simulink model "ProcessFlowRateModel_IMHRC2014v3"  (Simulink 7.9)
settings: Solver=VariableStepDiscrete  StartTime=0.0  StopTime=100.0  RelTol=1e-3
libraries: simeventslib x14
(part 2 of 2)

== system ProcessFlowRateModel_IMHRC2014v3/Pallet_STORE/Calculate_OUTFlow ==
  Calculate_OUTFlow : MATLAB Function  TreatAsAtomicUnit=on
  Entity Combiner : EntityCombiner  NumberInputPorts=2
  Entity Sink : EntitySink
  Entity Splitter : EntitySplitter  NumberOutputPorts=2
  FIFO Queue : FIFOQueue  Capacity=inf
  Get Attribute : GetAttribute  AttributeName=UoH|Quantity|OUTFlow  AttributeMissing=Error|Error|Error  AttributeDefaultValue=1|1|1  AttributeTreatAsVector=1|1|1  AttributeSendTiming=After entity departure|After entity departure|After entity departure  EvaluatedDefaultAttributeValue={[];[];[]}
      settings: OutputPortMap=o1,o2,o3
  Set Attribute : SetAttribute  AttributeName=OUTFlow  AttributeFrom=Signal port  EvaluatedAttributeValue={[]}
  Single Server : SingleServer  ServiceTime=0
  FlowRecord_IN : PMIOPort  Port=1  Side=Left
  FlowRecord_OUT : PMIOPort  Port=2  Side=Left
  OUTFlow_Signal : PMIOPort  Port=3  Side=Right
  wires:
  Get Attribute/1 -> Calculate_OUTFlow/1(UoH)
  Calculate_OUTFlow/1(OUTFlow_return) -> Set Attribute/1
  Get Attribute/2 -> Calculate_OUTFlow/2(Quantity)
  Get Attribute/3 -> Calculate_OUTFlow/3(OUTFlow)
  connections:
  Entity Combiner/RConn1 -- Get Attribute/LConn1
  Set Attribute/RConn1 -- Entity Splitter/LConn1
  Get Attribute/RConn1 -- Single Server/LConn1
  Single Server/RConn1 -- Set Attribute/LConn1
  FlowRecord_OUT/RConn1 -- Entity Splitter/RConn1
  FlowRecord_IN/RConn1 -- Entity Combiner/LConn1
  OUTFlow_Signal/RConn1 -- FIFO Queue/LConn1
  FIFO Queue/RConn1 -- Entity Combiner/LConn2
  Entity Splitter/RConn2 -- Entity Sink/LConn1

== system ProcessFlowRateModel_IMHRC2014v3/Pallet_STORE/FlowRecord ==
  Discrete Event Signal to Workspace : simeventslib/SimEvents Sinks/Discrete Event Signal to Workspace  VariableName=INFlow_Metric_PalletStore  SaveFormat=Structure With Time  isMonitorOnly=off  isRecordIC=off
  Discrete Event Signal to Workspace1 : simeventslib/SimEvents Sinks/Discrete Event Signal to Workspace  VariableName=OUTFlow_Metric_PalletStore  SaveFormat=Structure With Time  isMonitorOnly=off  isRecordIC=off
  FIFO Queue : FIFOQueue
  FlowRecord : TimeBasedFunctionCallGenerator  EventGenerationMode=Only at simulation start
  Get Attribute : GetAttribute  AttributeName=OUTFlow|INFlow  AttributeMissing=Error|Error  AttributeDefaultValue=1|1  AttributeTreatAsVector=1|1  AttributeSendTiming=After entity departure|After entity departure  EvaluatedDefaultAttributeValue={[];[]}
      settings: OutputPortMap=o1,o2
  Initialize_FlowRecord : SetAttribute  AttributeName=INFlow|OUTFlow  AttributeFrom=Dialog|Dialog  AttributeValue=[0 0 0 0 0]|[0 0 0 0 0]  AttributeTreatAsVector=1|1  EvaluatedAttributeValue={[0 0 0 0 0];[0 0 0 0 0]}
  New_FlowRecord : EventBasedEntityGenerator  GenerateEntitiesUpon=Function call from port fcn
  Output Switch : OutputSwitch  NumberOutputPorts=2
  Path Combiner1 : PathCombiner
  TO_INFlow : PMIOPort  Port=1  Side=Right
  TO_OUTFlow : PMIOPort  Port=2  Side=Left
  FROM_INFlow : PMIOPort  Port=3  Side=Right
  FROM_OUTFlow : PMIOPort  Port=4  Side=Left
  wires:
  FlowRecord/1 -> New_FlowRecord/1
  Get Attribute/2 -> Discrete Event Signal to Workspace/1
  Get Attribute/1 -> Discrete Event Signal to Workspace1/1
  connections:
  Output Switch/LConn1 -- FIFO Queue/RConn1
  New_FlowRecord/RConn1 -- Initialize_FlowRecord/LConn1
  Initialize_FlowRecord/RConn1 -- Path Combiner1/LConn1
  TO_INFlow/RConn1 -- Output Switch/RConn1
  TO_OUTFlow/RConn1 -- Output Switch/RConn2
  FROM_INFlow/RConn1 -- Path Combiner1/LConn2
  FROM_OUTFlow/RConn1 -- Path Combiner1/LConn3
  Path Combiner1/RConn1 -- Get Attribute/LConn1
  Get Attribute/RConn1 -- FIFO Queue/LConn1

== system ProcessFlowRateModel_IMHRC2014v3/Pallet_STORE/STORE ==
  Entity Sink : EntitySink
  FROM_STORE : Replicate  NumberOutputPorts=2
  InventoryRecord : Subsystem
  Message2Flow : Subsystem
  Message_Queue : FIFOQueue
  TO_STORE : Replicate  NumberOutputPorts=2
  Update_InventoryRecord_INFlow : Subsystem
  Update_InventoryRecord_OUTFlow : Subsystem
  Flow_IN : PMIOPort  Port=1  Side=Left
  Message_IN : PMIOPort  Port=2  Side=Left
  Flow_OUT : PMIOPort  Port=3  Side=Right
  Message_OUT : PMIOPort  Port=4  Side=Right
  connections:
  InventoryRecord/RConn1 -- Update_InventoryRecord_INFlow/RConn1
  Update_InventoryRecord_INFlow/RConn2 -- InventoryRecord/RConn2
  Flow_IN/RConn1 -- TO_STORE/LConn1
  TO_STORE/RConn1 -- Update_InventoryRecord_INFlow/LConn1
  TO_STORE/RConn2 -- Entity Sink/LConn1
  Message2Flow/RConn1 -- FROM_STORE/LConn1
  FROM_STORE/RConn2 -- Flow_OUT/RConn1
  Update_InventoryRecord_OUTFlow/LConn1 -- FROM_STORE/RConn1
  InventoryRecord/LConn1 -- Update_InventoryRecord_OUTFlow/RConn1
  InventoryRecord/LConn2 -- Update_InventoryRecord_OUTFlow/RConn2
  Message_IN/RConn1 -- Message_Queue/LConn1
  Message_Queue/RConn1 -- Message2Flow/LConn1

== system ProcessFlowRateModel_IMHRC2014v3/Parcel_OA/Calculate_INFlow ==
  Calculate_INFlow : MATLAB Function  TreatAsAtomicUnit=on
  Entity Combiner : EntityCombiner  NumberInputPorts=2
  Entity Sink : EntitySink
  Entity Splitter : EntitySplitter  NumberOutputPorts=2
  FIFO Queue : FIFOQueue  Capacity=inf
  Get Attribute : GetAttribute  AttributeName=UoH|Quantity|INFlow  AttributeMissing=Error|Error|Error  AttributeDefaultValue=1|1|1  AttributeTreatAsVector=1|1|1  AttributeSendTiming=After entity departure|After entity departure|After entity departure  EvaluatedDefaultAttributeValue={[];[];[]}
      settings: OutputPortMap=o1,o2,o3
  Set Attribute : SetAttribute  AttributeName=INFlow  AttributeFrom=Signal port  EvaluatedAttributeValue={[]}
  Single Server : SingleServer  ServiceTime=0
  FlowRecord_IN : PMIOPort  Port=1  Side=Right
  FlowRecord_OUT : PMIOPort  Port=2  Side=Right
  INFlow_Signal : PMIOPort  Port=3  Side=Left
  wires:
  Get Attribute/1 -> Calculate_INFlow/1(UoH)
  Calculate_INFlow/1(INFlow_return) -> Set Attribute/1
  Get Attribute/2 -> Calculate_INFlow/2(Quantity)
  Get Attribute/3 -> Calculate_INFlow/3(INFlow)
  connections:
  Entity Combiner/RConn1 -- Get Attribute/LConn1
  Set Attribute/RConn1 -- Entity Splitter/LConn1
  Get Attribute/RConn1 -- Single Server/LConn1
  Single Server/RConn1 -- Set Attribute/LConn1
  FlowRecord_OUT/RConn1 -- Entity Splitter/RConn1
  FlowRecord_IN/RConn1 -- Entity Combiner/LConn1
  Entity Splitter/RConn2 -- Entity Sink/LConn1
  INFlow_Signal/RConn1 -- FIFO Queue/LConn1
  FIFO Queue/RConn1 -- Entity Combiner/LConn2

== system ProcessFlowRateModel_IMHRC2014v3/Parcel_OA/Calculate_OUTFlow ==
  Calculate_OUTFlow : MATLAB Function  TreatAsAtomicUnit=on
  Entity Combiner : EntityCombiner  NumberInputPorts=2
  Entity Sink : EntitySink
  Entity Splitter : EntitySplitter  NumberOutputPorts=2
  FIFO Queue : FIFOQueue  Capacity=inf
  Get Attribute : GetAttribute  AttributeName=UoH|Quantity|OUTFlow  AttributeMissing=Error|Error|Error  AttributeDefaultValue=1|1|1  AttributeTreatAsVector=1|1|1  AttributeSendTiming=After entity departure|After entity departure|After entity departure  EvaluatedDefaultAttributeValue={[];[];[]}
      settings: OutputPortMap=o1,o2,o3
  Set Attribute : SetAttribute  AttributeName=OUTFlow  AttributeFrom=Signal port  EvaluatedAttributeValue={[]}
  Single Server : SingleServer  ServiceTime=0
  FlowRecord_IN : PMIOPort  Port=1  Side=Left
  FlowRecord_OUT : PMIOPort  Port=2  Side=Left
  OUTFlow_Signal : PMIOPort  Port=3  Side=Right
  wires:
  Get Attribute/1 -> Calculate_OUTFlow/1(UoH)
  Calculate_OUTFlow/1(OUTFlow_return) -> Set Attribute/1
  Get Attribute/2 -> Calculate_OUTFlow/2(Quantity)
  Get Attribute/3 -> Calculate_OUTFlow/3(OUTFlow)
  connections:
  Entity Combiner/RConn1 -- Get Attribute/LConn1
  Set Attribute/RConn1 -- Entity Splitter/LConn1
  Get Attribute/RConn1 -- Single Server/LConn1
  Single Server/RConn1 -- Set Attribute/LConn1
  FlowRecord_OUT/RConn1 -- Entity Splitter/RConn1
  FlowRecord_IN/RConn1 -- Entity Combiner/LConn1
  OUTFlow_Signal/RConn1 -- FIFO Queue/LConn1
  FIFO Queue/RConn1 -- Entity Combiner/LConn2
  Entity Splitter/RConn2 -- Entity Sink/LConn1

== system ProcessFlowRateModel_IMHRC2014v3/Parcel_OA/FRN_Process ==
  FIFO Queue1 : FIFOQueue
  N-Server : NServer  NumberOfServers=inf  ServiceTime=0
  Flow_IN : PMIOPort  Port=1  Side=Left
  Message_IN : PMIOPort  Port=2  Side=Left
  Flow_OUT : PMIOPort  Port=3  Side=Right
  Message_OUT : PMIOPort  Port=4  Side=Right
  connections:
  FIFO Queue1/RConn1 -- N-Server/LConn1
  Flow_IN/RConn1 -- FIFO Queue1/LConn1
  Flow_OUT/RConn1 -- N-Server/RConn1
  Message_OUT/RConn1 -- Message_IN/RConn1

== system ProcessFlowRateModel_IMHRC2014v3/Parcel_OA/FlowRecord ==
  Discrete Event Signal to Workspace : simeventslib/SimEvents Sinks/Discrete Event Signal to Workspace  VariableName=INFlow_Metric  SaveFormat=Structure With Time  isMonitorOnly=off  isRecordIC=off
  Discrete Event Signal to Workspace1 : simeventslib/SimEvents Sinks/Discrete Event Signal to Workspace  VariableName=OUTFlow_Metric  SaveFormat=Structure With Time  isMonitorOnly=off  isRecordIC=off
  FIFO Queue : FIFOQueue
  FlowRecord : TimeBasedFunctionCallGenerator  EventGenerationMode=Only at simulation start
  Get Attribute : GetAttribute  AttributeName=OUTFlow|INFlow  AttributeMissing=Error|Error  AttributeDefaultValue=1|1  AttributeTreatAsVector=1|1  AttributeSendTiming=After entity departure|After entity departure  EvaluatedDefaultAttributeValue={[];[]}
      settings: OutputPortMap=o1,o2
  Initialize_FlowRecord : SetAttribute  AttributeName=INFlow|OUTFlow  AttributeFrom=Dialog|Dialog  AttributeValue=[0 0 0 0 0]|[0 0 0 0 0]  AttributeTreatAsVector=1|1  EvaluatedAttributeValue={[0 0 0 0 0];[0 0 0 0 0]}
  New_FlowRecord : EventBasedEntityGenerator  GenerateEntitiesUpon=Function call from port fcn
  Output Switch : OutputSwitch  NumberOutputPorts=2
  Path Combiner1 : PathCombiner
  TO_INFlow : PMIOPort  Port=1  Side=Right
  TO_OUTFlow : PMIOPort  Port=2  Side=Left
  FROM_INFlow : PMIOPort  Port=3  Side=Right
  FROM_OUTFlow : PMIOPort  Port=4  Side=Left
  wires:
  FlowRecord/1 -> New_FlowRecord/1
  Get Attribute/2 -> Discrete Event Signal to Workspace/1
  Get Attribute/1 -> Discrete Event Signal to Workspace1/1
  connections:
  Output Switch/LConn1 -- FIFO Queue/RConn1
  New_FlowRecord/RConn1 -- Initialize_FlowRecord/LConn1
  Initialize_FlowRecord/RConn1 -- Path Combiner1/LConn1
  TO_INFlow/RConn1 -- Output Switch/RConn1
  TO_OUTFlow/RConn1 -- Output Switch/RConn2
  FROM_INFlow/RConn1 -- Path Combiner1/LConn2
  FROM_OUTFlow/RConn1 -- Path Combiner1/LConn3
  Path Combiner1/RConn1 -- Get Attribute/LConn1
  Get Attribute/RConn1 -- FIFO Queue/LConn1

== system ProcessFlowRateModel_IMHRC2014v3/Parcel_SHIP/OrderFamily_Parcel_SOURCE ==
  Carton_Quantity1 : EventBasedRandomNumber  Distribution=Discrete uniform  minUnid=1  maxUnid=15  numValueUnid=15  valueVecDisc=[1 2 3]  probVecDisc=[0.5 0.35 0.15]  Seed=38014
  Pallet_Source1 : TimeBasedEntityGenerator
  Set_Pallet1 : SetAttribute  AttributeName=UoH|CartonQuantity|Quantity  AttributeFrom=Dialog|Signal port|Dialog  AttributeValue=1|1|1  AttributeTreatAsVector=1|1|1  EvaluatedAttributeValue={1;[];1}
      settings: InputPortMap=u1
  Conn1 : PMIOPort  Port=1  Side=Right
  wires:
  Carton_Quantity1/1 -> Set_Pallet1/1
  connections:
  Pallet_Source1/RConn1 -- Set_Pallet1/LConn1
  Conn1/RConn1 -- Set_Pallet1/RConn1

== system ProcessFlowRateModel_IMHRC2014v3/Each_STORE/STORE/InventoryRecord ==
  Discrete Event Signal to Workspace : simeventslib/SimEvents Sinks/Discrete Event Signal to Workspace  VariableName=Net_Inventory_PalletStore  SaveFormat=Structure With Time  isMonitorOnly=off  isRecordIC=off
  FIFO Queue : FIFOQueue
  Get Attribute : GetAttribute  AttributeName=Net_Inventory  EvaluatedDefaultAttributeValue={[]}
      settings: OutputPortMap=o1
  Initialize_FlowRecord : SetAttribute  AttributeName=Net_Inventory  AttributeValue=[0 0 0 0 0]  EvaluatedAttributeValue={[0 0 0 0 0]}
  InventoryRecord : TimeBasedFunctionCallGenerator  EventGenerationMode=Only at simulation start
  New_InventoryRecord : EventBasedEntityGenerator  GenerateEntitiesUpon=Function call from port fcn
  Output Switch : OutputSwitch  NumberOutputPorts=2
  Path Combiner : PathCombiner
  TO_INFlow : PMIOPort  Port=1  Side=Right
  TO_OUTFlow : PMIOPort  Port=2  Side=Left
  FROM_INFlow : PMIOPort  Port=3  Side=Right
  FROM_OUTFlow : PMIOPort  Port=4  Side=Left
  wires:
  InventoryRecord/1 -> New_InventoryRecord/1
  Get Attribute/1 -> Discrete Event Signal to Workspace/1
  connections:
  Output Switch/LConn1 -- FIFO Queue/RConn1
  New_InventoryRecord/RConn1 -- Initialize_FlowRecord/LConn1
  Initialize_FlowRecord/RConn1 -- Path Combiner/LConn1
  TO_INFlow/RConn1 -- Output Switch/RConn1
  TO_OUTFlow/RConn1 -- Output Switch/RConn2
  FROM_INFlow/RConn1 -- Path Combiner/LConn2
  FROM_OUTFlow/RConn1 -- Path Combiner/LConn3
  Path Combiner/RConn1 -- Get Attribute/LConn1
  Get Attribute/RConn1 -- FIFO Queue/LConn1

== system ProcessFlowRateModel_IMHRC2014v3/Each_STORE/STORE/Message2Flow ==
  Entity Departure Function-Call Generator : EntityDepartureFunctionCallGenerator
  Generate_Flow_Entity : EventBasedEntityGenerator  GenerateEntitiesUpon=Function call from port fcn
  Get_Order_Attribute : GetAttribute  AttributeName=UoH|Quantity  AttributeMissing=Error|Error  AttributeDefaultValue=1|1  AttributeTreatAsVector=1|1  AttributeSendTiming=After entity departure|After entity departure  EvaluatedDefaultAttributeValue={[];[]}
      settings: OutputPortMap=o1,o2
  Message_Sink : EntitySink
  Set_Flow_Attribute : SetAttribute  AttributeName=UoH|Quantity  AttributeFrom=Signal port|Signal port  AttributeValue=1|1  AttributeTreatAsVector=1|1  EvaluatedAttributeValue={[];[]}
      settings: InputPortMap=u0,u1
  Single Server : SingleServer  ServiceTime=0
  Message_IN : PMIOPort  Port=1  Side=Left
  Flow_OUT : PMIOPort  Port=2  Side=Right
  wires:
  Entity Departure Function-Call Generator/1 -> Generate_Flow_Entity/1
  Get_Order_Attribute/1 -> Set_Flow_Attribute/1
  Get_Order_Attribute/2 -> Set_Flow_Attribute/2
  connections:
  Get_Order_Attribute/RConn1 -- Entity Departure Function-Call Generator/LConn1
  Entity Departure Function-Call Generator/RConn1 -- Message_Sink/LConn1
  Generate_Flow_Entity/RConn1 -- Single Server/LConn1
  Single Server/RConn1 -- Set_Flow_Attribute/LConn1
  Message_IN/RConn1 -- Get_Order_Attribute/LConn1
  Flow_OUT/RConn1 -- Set_Flow_Attribute/RConn1

== system ProcessFlowRateModel_IMHRC2014v3/Each_STORE/STORE/Update_InventoryRecord_INFlow ==
  Calculate_Inventory : MATLAB Function  TreatAsAtomicUnit=on
  Entity Combiner : EntityCombiner  NumberInputPorts=2
  Entity Sink : EntitySink
  Entity Splitter : EntitySplitter  NumberOutputPorts=2
  FIFO Queue : FIFOQueue  Capacity=inf
  Get Attribute : GetAttribute  AttributeName=UoH|Quantity|Net_Inventory  AttributeMissing=Error|Error|Error  AttributeDefaultValue=1|1|1  AttributeTreatAsVector=1|1|1  AttributeSendTiming=After entity departure|After entity departure|After entity departure  EvaluatedDefaultAttributeValue={[];[];[]}
      settings: OutputPortMap=o1,o2,o3
  Set Attribute : SetAttribute  AttributeName=Net_Inventory  AttributeFrom=Signal port  EvaluatedAttributeValue={[]}
  Single Server : SingleServer  ServiceTime=0
  InventoryRecord_IN : PMIOPort  Port=1  Side=Right
  InventoryRecord_OUT : PMIOPort  Port=2  Side=Right
  Signal_IN : PMIOPort  Port=3  Side=Left
  wires:
  Get Attribute/1 -> Calculate_Inventory/1(UoH)
  Calculate_Inventory/1(Net_Inventory1) -> Set Attribute/1
  Get Attribute/2 -> Calculate_Inventory/2(Quantity)
  Get Attribute/3 -> Calculate_Inventory/3(Net_Inventory)
  connections:
  Entity Combiner/RConn1 -- Get Attribute/LConn1
  Set Attribute/RConn1 -- Entity Splitter/LConn1
  Get Attribute/RConn1 -- Single Server/LConn1
  Single Server/RConn1 -- Set Attribute/LConn1
  InventoryRecord_OUT/RConn1 -- Entity Splitter/RConn1
  InventoryRecord_IN/RConn1 -- Entity Combiner/LConn1
  Entity Splitter/RConn2 -- Entity Sink/LConn1
  Signal_IN/RConn1 -- FIFO Queue/LConn1
  FIFO Queue/RConn1 -- Entity Combiner/LConn2

== system ProcessFlowRateModel_IMHRC2014v3/Each_STORE/STORE/Update_InventoryRecord_OUTFlow ==
  Calculate_Inventory : MATLAB Function  TreatAsAtomicUnit=on
  Entity Combiner : EntityCombiner  NumberInputPorts=2
  Entity Sink : EntitySink
  Entity Splitter : EntitySplitter  NumberOutputPorts=2
  FIFO Queue : FIFOQueue  Capacity=inf
  Get Attribute : GetAttribute  AttributeName=UoH|Quantity|Net_Inventory  AttributeMissing=Error|Error|Error  AttributeDefaultValue=1|1|1  AttributeTreatAsVector=1|1|1  AttributeSendTiming=After entity departure|After entity departure|After entity departure  EvaluatedDefaultAttributeValue={[];[];[]}
      settings: OutputPortMap=o1,o2,o3
  Set Attribute : SetAttribute  AttributeName=Net_Inventory  AttributeFrom=Signal port  EvaluatedAttributeValue={[]}
  Single Server : SingleServer  ServiceTime=0
  InventoryRecord_IN : PMIOPort  Port=1  Side=Right
  InventoryRecord_OUT : PMIOPort  Port=2  Side=Right
  Signal_IN : PMIOPort  Port=3  Side=Left
  wires:
  Get Attribute/1 -> Calculate_Inventory/1(UoH)
  Calculate_Inventory/1(Net_Inventory1) -> Set Attribute/1
  Get Attribute/2 -> Calculate_Inventory/2(Quantity)
  Get Attribute/3 -> Calculate_Inventory/3(Net_Inventory)
  connections:
  Entity Combiner/RConn1 -- Get Attribute/LConn1
  Set Attribute/RConn1 -- Entity Splitter/LConn1
  Get Attribute/RConn1 -- Single Server/LConn1
  Single Server/RConn1 -- Set Attribute/LConn1
  InventoryRecord_OUT/RConn1 -- Entity Splitter/RConn1
  InventoryRecord_IN/RConn1 -- Entity Combiner/LConn1
  Entity Splitter/RConn2 -- Entity Sink/LConn1
  Signal_IN/RConn1 -- FIFO Queue/LConn1
  FIFO Queue/RConn1 -- Entity Combiner/LConn2

== system ProcessFlowRateModel_IMHRC2014v3/Pallet_STORE/STORE/InventoryRecord ==
  Discrete Event Signal to Workspace : simeventslib/SimEvents Sinks/Discrete Event Signal to Workspace  VariableName=Net_Inventory_PalletStore  SaveFormat=Structure With Time  isMonitorOnly=off  isRecordIC=off
  FIFO Queue : FIFOQueue
  Get Attribute : GetAttribute  AttributeName=Net_Inventory  EvaluatedDefaultAttributeValue={[]}
      settings: OutputPortMap=o1
  Initialize_FlowRecord : SetAttribute  AttributeName=Net_Inventory  AttributeValue=[0 0 0 0 0]  EvaluatedAttributeValue={[0 0 0 0 0]}
  InventoryRecord : TimeBasedFunctionCallGenerator  EventGenerationMode=Only at simulation start
  New_InventoryRecord : EventBasedEntityGenerator  GenerateEntitiesUpon=Function call from port fcn
  Output Switch : OutputSwitch  NumberOutputPorts=2
  Path Combiner : PathCombiner
  TO_INFlow : PMIOPort  Port=1  Side=Right
  TO_OUTFlow : PMIOPort  Port=2  Side=Left
  FROM_INFlow : PMIOPort  Port=3  Side=Right
  FROM_OUTFlow : PMIOPort  Port=4  Side=Left
  wires:
  InventoryRecord/1 -> New_InventoryRecord/1
  Get Attribute/1 -> Discrete Event Signal to Workspace/1
  connections:
  Output Switch/LConn1 -- FIFO Queue/RConn1
  New_InventoryRecord/RConn1 -- Initialize_FlowRecord/LConn1
  Initialize_FlowRecord/RConn1 -- Path Combiner/LConn1
  TO_INFlow/RConn1 -- Output Switch/RConn1
  TO_OUTFlow/RConn1 -- Output Switch/RConn2
  FROM_INFlow/RConn1 -- Path Combiner/LConn2
  FROM_OUTFlow/RConn1 -- Path Combiner/LConn3
  Path Combiner/RConn1 -- Get Attribute/LConn1
  Get Attribute/RConn1 -- FIFO Queue/LConn1

== system ProcessFlowRateModel_IMHRC2014v3/Pallet_STORE/STORE/Message2Flow ==
  Entity Departure Function-Call Generator : EntityDepartureFunctionCallGenerator
  Generate_Flow_Entity : EventBasedEntityGenerator  GenerateEntitiesUpon=Function call from port fcn
  Get_Order_Attribute : GetAttribute  AttributeName=UoH|Quantity  AttributeMissing=Error|Error  AttributeDefaultValue=1|1  AttributeTreatAsVector=1|1  AttributeSendTiming=After entity departure|After entity departure  EvaluatedDefaultAttributeValue={[];[]}
      settings: OutputPortMap=o1,o2
  Message_Sink : EntitySink
  Set_Flow_Attribute : SetAttribute  AttributeName=UoH|Quantity  AttributeFrom=Signal port|Signal port  AttributeValue=1|1  AttributeTreatAsVector=1|1  EvaluatedAttributeValue={[];[]}
      settings: InputPortMap=u0,u1
  Single Server : SingleServer  ServiceTime=0
  Message_IN : PMIOPort  Port=1  Side=Left
  Flow_OUT : PMIOPort  Port=2  Side=Right
  wires:
  Entity Departure Function-Call Generator/1 -> Generate_Flow_Entity/1
  Get_Order_Attribute/1 -> Set_Flow_Attribute/1
  Get_Order_Attribute/2 -> Set_Flow_Attribute/2
  connections:
  Get_Order_Attribute/RConn1 -- Entity Departure Function-Call Generator/LConn1
  Entity Departure Function-Call Generator/RConn1 -- Message_Sink/LConn1
  Generate_Flow_Entity/RConn1 -- Single Server/LConn1
  Single Server/RConn1 -- Set_Flow_Attribute/LConn1
  Message_IN/RConn1 -- Get_Order_Attribute/LConn1
  Flow_OUT/RConn1 -- Set_Flow_Attribute/RConn1

== system ProcessFlowRateModel_IMHRC2014v3/Pallet_STORE/STORE/Update_InventoryRecord_INFlow ==
  Calculate_Inventory : MATLAB Function  TreatAsAtomicUnit=on
  Entity Combiner : EntityCombiner  NumberInputPorts=2
  Entity Sink : EntitySink
  Entity Splitter : EntitySplitter  NumberOutputPorts=2
  FIFO Queue : FIFOQueue  Capacity=inf
  Get Attribute : GetAttribute  AttributeName=UoH|Quantity|Net_Inventory  AttributeMissing=Error|Error|Error  AttributeDefaultValue=1|1|1  AttributeTreatAsVector=1|1|1  AttributeSendTiming=After entity departure|After entity departure|After entity departure  EvaluatedDefaultAttributeValue={[];[];[]}
      settings: OutputPortMap=o1,o2,o3
  Set Attribute : SetAttribute  AttributeName=Net_Inventory  AttributeFrom=Signal port  EvaluatedAttributeValue={[]}
  Single Server : SingleServer  ServiceTime=0
  InventoryRecord_IN : PMIOPort  Port=1  Side=Right
  InventoryRecord_OUT : PMIOPort  Port=2  Side=Right
  Signal_IN : PMIOPort  Port=3  Side=Left
  wires:
  Get Attribute/1 -> Calculate_Inventory/1(UoH)
  Calculate_Inventory/1(Net_Inventory1) -> Set Attribute/1
  Get Attribute/2 -> Calculate_Inventory/2(Quantity)
  Get Attribute/3 -> Calculate_Inventory/3(Net_Inventory)
  connections:
  Entity Combiner/RConn1 -- Get Attribute/LConn1
  Set Attribute/RConn1 -- Entity Splitter/LConn1
  Get Attribute/RConn1 -- Single Server/LConn1
  Single Server/RConn1 -- Set Attribute/LConn1
  InventoryRecord_OUT/RConn1 -- Entity Splitter/RConn1
  InventoryRecord_IN/RConn1 -- Entity Combiner/LConn1
  Entity Splitter/RConn2 -- Entity Sink/LConn1
  Signal_IN/RConn1 -- FIFO Queue/LConn1
  FIFO Queue/RConn1 -- Entity Combiner/LConn2

== system ProcessFlowRateModel_IMHRC2014v3/Pallet_STORE/STORE/Update_InventoryRecord_OUTFlow ==
  Calculate_Inventory : MATLAB Function  TreatAsAtomicUnit=on
  Entity Combiner : EntityCombiner  NumberInputPorts=2
  Entity Sink : EntitySink
  Entity Splitter : EntitySplitter  NumberOutputPorts=2
  FIFO Queue : FIFOQueue  Capacity=inf
  Get Attribute : GetAttribute  AttributeName=UoH|Quantity|Net_Inventory  AttributeMissing=Error|Error|Error  AttributeDefaultValue=1|1|1  AttributeTreatAsVector=1|1|1  AttributeSendTiming=After entity departure|After entity departure|After entity departure  EvaluatedDefaultAttributeValue={[];[];[]}
      settings: OutputPortMap=o1,o2,o3
  Set Attribute : SetAttribute  AttributeName=Net_Inventory  AttributeFrom=Signal port  EvaluatedAttributeValue={[]}
  Single Server : SingleServer  ServiceTime=0
  InventoryRecord_IN : PMIOPort  Port=1  Side=Right
  InventoryRecord_OUT : PMIOPort  Port=2  Side=Right
  Signal_IN : PMIOPort  Port=3  Side=Left
  wires:
  Get Attribute/1 -> Calculate_Inventory/1(UoH)
  Calculate_Inventory/1(Net_Inventory1) -> Set Attribute/1
  Get Attribute/2 -> Calculate_Inventory/2(Quantity)
  Get Attribute/3 -> Calculate_Inventory/3(Net_Inventory)
  connections:
  Entity Combiner/RConn1 -- Get Attribute/LConn1
  Set Attribute/RConn1 -- Entity Splitter/LConn1
  Get Attribute/RConn1 -- Single Server/LConn1
  Single Server/RConn1 -- Set Attribute/LConn1
  InventoryRecord_OUT/RConn1 -- Entity Splitter/RConn1
  InventoryRecord_IN/RConn1 -- Entity Combiner/LConn1
  Entity Splitter/RConn2 -- Entity Sink/LConn1
  Signal_IN/RConn1 -- FIFO Queue/LConn1
  FIFO Queue/RConn1 -- Entity Combiner/LConn2

== matlab function LTL_OA/Calculate_INFlow/Calculate_INFlow ==
  data: UoH input double; INFlow_return output double; Quantity input double; INFlow input double
function INFlow_return  = Calculate_INFlow(UoH, Quantity, INFlow)
%#codegen

INFlow_return = INFlow;


if eq(UoH, 0) == 0
%test if parameters are initialized

    INFlow_return(UoH) = INFlow(UoH) + Quantity;
end

== matlab function LTL_OA/Calculate_OUTFlow/Calculate_OUTFlow ==
  data: UoH input double; OUTFlow_return output double; Quantity input double; OUTFlow input double
function OUTFlow_return  = Calculate_OUTFlow(UoH, Quantity, OUTFlow)
%#codegen

OUTFlow_return = OUTFlow;


if eq(UoH, 0) == 0
%test if parameters are initialized

    OUTFlow_return(UoH) = OUTFlow(UoH) + Quantity;
end

== matlab function Pallet_STORE/Calculate_INFlow/Calculate_INFlow ==
  data: UoH input double; INFlow_return output double; Quantity input double; INFlow input double
function INFlow_return  = Calculate_INFlow(UoH, Quantity, INFlow)
%#codegen

INFlow_return = INFlow;


if eq(UoH, 0) == 0
%test if parameters are initialized

    INFlow_return(UoH) = INFlow(UoH) + Quantity;
end

== matlab function Pallet_STORE/Calculate_OUTFlow/Calculate_OUTFlow ==
  data: UoH input double; OUTFlow_return output double; Quantity input double; OUTFlow input double
function OUTFlow_return  = Calculate_OUTFlow(UoH, Quantity, OUTFlow)
%#codegen

OUTFlow_return = OUTFlow;


if eq(UoH, 0) == 0
%test if parameters are initialized

    OUTFlow_return(UoH) = OUTFlow(UoH) + Quantity;
end

== matlab function Pallet_STORE/STORE/Update_InventoryRecord_INFlow/Calculate_Inventory ==
  data: UoH input double; Quantity input double; Net_Inventory input double; Net_Inventory1 output double
function Net_Inventory1  = Calculate_INFlow(UoH, Quantity, Net_Inventory)
%#codegen

Net_Inventory1 = Net_Inventory;


if eq(UoH, 0) == 0
%test if parameters are initialized

    Net_Inventory1(UoH) = Net_Inventory(UoH) + Quantity;
end

== matlab function Pallet_STORE/STORE/Update_InventoryRecord_OUTFlow/Calculate_Inventory ==
  data: UoH input double; Quantity input double; Net_Inventory input double; Net_Inventory1 output double
function Net_Inventory1  = Calculate_INFlow(UoH, Quantity, Net_Inventory)
%#codegen

Net_Inventory1 = Net_Inventory;


if eq(UoH, 0) == 0
%test if parameters are initialized

    Net_Inventory1(UoH) = Net_Inventory(UoH) - Quantity;
end

== matlab function MixedPallet_Assy/Calculate_INFlow/Calculate_INFlow ==
  data: UoH input double; INFlow_return output double; Quantity input double; INFlow input double
function INFlow_return  = Calculate_INFlow(UoH, Quantity, INFlow)
%#codegen

INFlow_return = INFlow;


if eq(UoH, 0) == 0
%test if parameters are initialized

    INFlow_return(UoH) = INFlow(UoH) + Quantity;
end

== matlab function MixedPallet_Assy/Calculate_OUTFlow/Calculate_OUTFlow ==
  data: UoH input double; OUTFlow_return output double; Quantity input double; OUTFlow input double
function OUTFlow_return  = Calculate_OUTFlow(UoH, Quantity, OUTFlow)
%#codegen

OUTFlow_return = OUTFlow;


if eq(UoH, 0) == 0
%test if parameters are initialized

    OUTFlow_return(UoH) = OUTFlow(UoH) + Quantity;
end

== matlab function Parcel_OA/Calculate_INFlow/Calculate_INFlow ==
  data: UoH input double; INFlow_return output double; Quantity input double; INFlow input double
function INFlow_return  = Calculate_INFlow(UoH, Quantity, INFlow)
%#codegen

INFlow_return = INFlow;


if eq(UoH, 0) == 0
%test if parameters are initialized

    INFlow_return(UoH) = INFlow(UoH) + Quantity;
end

== matlab function Parcel_OA/Calculate_OUTFlow/Calculate_OUTFlow ==
  data: UoH input double; OUTFlow_return output double; Quantity input double; OUTFlow input double
function OUTFlow_return  = Calculate_OUTFlow(UoH, Quantity, OUTFlow)
%#codegen

OUTFlow_return = OUTFlow;


if eq(UoH, 0) == 0
%test if parameters are initialized

    OUTFlow_return(UoH) = OUTFlow(UoH) + Quantity;
end

== matlab function Each_STORE/Calculate_INFlow/Calculate_INFlow ==
  data: UoH input double; INFlow_return output double; Quantity input double; INFlow input double
function INFlow_return  = Calculate_INFlow(UoH, Quantity, INFlow)
%#codegen

INFlow_return = INFlow;


if eq(UoH, 0) == 0
%test if parameters are initialized

    INFlow_return(UoH) = INFlow(UoH) + Quantity;
end

== matlab function Each_STORE/Calculate_OUTFlow/Calculate_OUTFlow ==
  data: UoH input double; OUTFlow_return output double; Quantity input double; OUTFlow input double
function OUTFlow_return  = Calculate_OUTFlow(UoH, Quantity, OUTFlow)
%#codegen

OUTFlow_return = OUTFlow;


if eq(UoH, 0) == 0
%test if parameters are initialized

    OUTFlow_return(UoH) = OUTFlow(UoH) + Quantity;
end

== matlab function Each_STORE/STORE/Update_InventoryRecord_INFlow/Calculate_Inventory ==
  data: UoH input double; Quantity input double; Net_Inventory input double; Net_Inventory1 output double
function Net_Inventory1  = Calculate_INFlow(UoH, Quantity, Net_Inventory)
%#codegen

Net_Inventory1 = Net_Inventory;


if eq(UoH, 0) == 0
%test if parameters are initialized

    Net_Inventory1(UoH) = Net_Inventory(UoH) + Quantity;
end

== matlab function Each_STORE/STORE/Update_InventoryRecord_OUTFlow/Calculate_Inventory ==
  data: UoH input double; Quantity input double; Net_Inventory input double; Net_Inventory1 output double
function Net_Inventory1  = Calculate_INFlow(UoH, Quantity, Net_Inventory)
%#codegen

Net_Inventory1 = Net_Inventory;


if eq(UoH, 0) == 0
%test if parameters are initialized

    Net_Inventory1(UoH) = Net_Inventory(UoH) - Quantity;
end

== matlab function MixedCarton_Assy/Calculate_INFlow/Calculate_INFlow ==
  data: UoH input double; INFlow_return output double; Quantity input double; INFlow input double
function INFlow_return  = Calculate_INFlow(UoH, Quantity, INFlow)
%#codegen

INFlow_return = INFlow;


if eq(UoH, 0) == 0
%test if parameters are initialized

    INFlow_return(UoH) = INFlow(UoH) + Quantity;
end

== matlab function MixedCarton_Assy/Calculate_OUTFlow/Calculate_OUTFlow ==
  data: UoH input double; OUTFlow_return output double; Quantity input double; OUTFlow input double
function OUTFlow_return  = Calculate_OUTFlow(UoH, Quantity, OUTFlow)
%#codegen

OUTFlow_return = OUTFlow;


if eq(UoH, 0) == 0
%test if parameters are initialized

    OUTFlow_return(UoH) = OUTFlow(UoH) + Quantity;
end
